simulink model "SistemaCompleto_PMSM"  (R2023b)
settings: Solver=VariableStepAuto  StartTime=0.0  StopTime=2  RelTol=1e-3
PostLoadFcn:
  | parametros_sistema_completo
  | run("parametros_sistema_completo.mlx")
values from neighbouring files (symbols this model uses):
  a_cu = 3.9e-3    (= 0.0039)    [parametros_sistema_completo.m]    (also in workspace_params.mat)
  A_i = [0,  1,                          0 ... (first row only)    [analisis_estabilidad_LA.m]
  b_eq = params.b_total    [calcular_matriz_AO.m]    (also in calculo_incertidumbre_y_control.m = b_m + b_l/(r^2); parametros_sistema_completo.m = 2.19444444444e-05; workspace_params.mat = 2.19444444444e-05)
  C_ts = C_ts * (1 + tol_pct)    [calculo_incertidumbre_y_control.m]    (also in parametros_sistema_completo.m = 0.818; workspace_params.mat = 0.818)
  g = 9.80665    [parametros_sistema_completo.m]    (also in workspace_params.mat)
  J_eq = params.J_total    [calcular_matriz_AO.m]    (also in calculo_incertidumbre_y_control.m = J_m + J_l/r^2; parametros_sistema_completo.m = 1.97847222222e-05; workspace_params.mat = 3.28055555556e-05)
  k_l = m*l_cm + m_l*l_l    [calculo_incertidumbre_y_control.m]    (also in parametros_sistema_completo.m = 0.25; workspace_params.mat = 0.625)
  L_d = L_d    * (1 - tol_pct)    [calculo_incertidumbre_y_control.m]    (also in parametros_sistema_completo.m = 0.0066; workspace_params.mat = 0.0066)
  L_ls = L_ls   * (1 - tol_pct)    [calculo_incertidumbre_y_control.m]    (also in parametros_sistema_completo.m = 0.0008; workspace_params.mat = 0.0008)
  L_q = L_q    * (1 - tol_pct)    [calculo_incertidumbre_y_control.m]    (also in parametros_sistema_completo.m = 0.0058; workspace_params.mat = 0.0058)
  lambda_r = lambda_r * (1 + tol_pct)    [calculo_incertidumbre_y_control.m]    (also in parametros_sistema_completo.m = 0.016; workspace_params.mat = 0.016)
  P_p = 3    [parametros_sistema_completo.m]    (also in workspace_params.mat)
  params = struct()    [evaluar_migracion_Ids.m]    (also in parametros_sistema_completo.m; workspace_params.mat = )
  r = params.r_red    [calcular_matriz_AO.m]    (also in parametros_sistema_completo.m = 120; workspace_params.mat = 120)
  R_s_sim = R_sREF * (1 + a_cu * (T_s_sim - T_sREF))    [configurar_temperatura_516.m]
  R_sREF = R_sREF * (1 - tol_pct)    [calculo_incertidumbre_y_control.m]    (also in parametros_sistema_completo.m = 1.02; workspace_params.mat = 1.02)
  R_ts_amb = R_ts_amb * (1 - tol_pct)    [calculo_incertidumbre_y_control.m]    (also in parametros_sistema_completo.m = 146.7; workspace_params.mat = 146.7)
  T_amb = 20    [parametros_sistema_completo.m]    (also in workspace_params.mat)
  T_s = x(6)    [modulador_torque_521.m]    (also in simulacion_dinamica_516.m)
  T_sREF = 20    [parametros_sistema_completo.m]    (also in workspace_params.mat)
undefined symbols (not defined in the file or in its folder): A_T, A_theta, A_v, b_a, B_i, B_T, B_theta, B_v, C_i, C_T, C_theta, C_v, consigna_posicion, D_i, D_T, D_theta, D_v, i_ds_inicial, Is_pico, Is_rms_max, Is_rms_nom, K_e_i_m_int, K_e_tita_m, K_e_tita_m_int, K_e_w_m, K_e_w_m_int, K_p0, K_pd, K_pq, K_sa, K_sia, pos_inicial, t_rampa_acel, t_rampa_vel, V_sl_max, x0_ias, x0_ibs, x0_ics, x0_T, x0_theta
libraries: simulink_extras x8, SignalEditorBlockLib x6, eeStairGenerator x4, simulink x1
(part 4 of 7)

== system SistemaCompleto_PMSM/Modelo Global NL perfil trapezoidal aceleracion1/Controlador PID de Posicion ==
  ωm[rad/s] : Inport
  ωm*[rad/s] : Inport  Port=2
  Integrator : Integrator
  Integrator1 : Integrator
  K_sa : Gain  Gain=K_sa
  K_sia : Gain  Gain=K_sia
  Sum : Sum  Inputs=+++
  Sum1 : Sum  Inputs=-+|
  b_a : Gain  Gain=b_a
  Tm*' : Outport
  wires:
  K_sa/1 -> Sum/2
  K_sia/1 -> Sum/3
  Integrator1/1 -> Integrator/1, K_sa/1  "eθm"
  b_a/1 -> Sum/1
  Integrator/1 -> K_sia/1  "eθ/s"
  ωm[rad/s]/1 -> Sum1/1
  ωm*[rad/s]/1 -> Sum1/2
  Sum1/1 -> b_a/1, Integrator1/1  "eωm"
  Sum/1 -> Tm*'/1  "Tm*'"

== system SistemaCompleto_PMSM/Modelo Global NL perfil trapezoidal aceleracion1/Desacople de Realimentaciones Fisicas Naturales ==
  R_s : Inport
  ωm : Inport  Port=2
  i_qs : Inport  Port=3
  v_qs* : Inport  Port=4
  v_ds* : Inport  Port=5
  v_0s* : Inport  Port=6
  i_0s : Inport  Port=7
  i_ds : Inport  Port=8
  Constant : Constant  Value=lambda_r
  Gain : Gain  Gain=P_p
  Gain3 : Gain  Gain=L_q*P_p
  Gain4 : Gain  Gain=L_d
  Product{,1..4} (5 alike) : Product
  Sum : Sum  Inputs=|++
  Sum1 : Sum  Inputs=+++
  Sum2 : Sum  Inputs=+-+
  Sum3 : Sum  Inputs=++|
  v_qs [V] : Outport
  v_ds [V] : Outport  Port=2
  v_0s [V] : Outport  Port=3
  wires:
  i_ds/1 -> Product3/1, Gain4/1
  Product1/1 -> Sum1/3
  Gain/1 -> Sum1/2
  v_qs*/1 -> Sum1/1
  R_s/1 -> Product1/2, Product3/2, Product4/1
  i_qs/1 -> Product2/2, Product1/1
  Sum1/1 -> v_qs [V]/1  "v_qs [V]"
  Gain3/1 -> Sum2/2
  Product2/1 -> Gain3/1
  Product3/1 -> Sum2/3
  v_ds*/1 -> Sum2/1
  Sum2/1 -> v_ds [V]/1  "v_ds [V]"
  i_0s/1 -> Product4/2
  Product4/1 -> Sum3/2
  v_0s*/1 -> Sum3/1
  Sum3/1 -> v_0s [V]/1
  ωm/1 -> Product/1, Product2/1
  Constant/1 -> Sum/1
  Gain4/1 -> Sum/2
  Sum/1 -> Product/2
  Product/1 -> Gain/1

== system SistemaCompleto_PMSM/Modelo Global NL perfil trapezoidal aceleracion1/Modulador de Corriente ==
  i_qs : Inport
  i_qs* : Inport  Port=2
  i_ds* : Inport  Port=3
  i_ds : Inport  Port=4
  i_0s* : Inport  Port=5
  i_0s : Inport  Port=6
  Gain : Gain  Gain=K_pq
  K_p0 : Gain  Gain=K_p0
  K_pd : Gain  Gain=K_pd
  Sum : Sum  Inputs=|+-
  Sum1 : Sum  Inputs=|+-
  Sum2 : Sum  Inputs=|+-
  v_qs* : Outport
  v_ds* : Outport  Port=2
  v_0s* : Outport  Port=3
  wires:
  i_qs*/1 -> Sum/1
  K_pd/1 -> v_ds*/1
  i_0s*/1 -> Sum2/1
  Sum/1 -> Gain/1
  i_qs/1 -> Sum/2
  K_p0/1 -> v_0s*/1
  Sum1/1 -> K_pd/1
  Sum2/1 -> K_p0/1
  Gain/1 -> v_qs*/1
  i_ds*/1 -> Sum1/1
  i_ds/1 -> Sum1/2
  i_0s/1 -> Sum2/2

== system SistemaCompleto_PMSM/Modelo Global NL perfil trapezoidal aceleracion1/Modulador de Tensión no ideal espacio de estados ==
  V_c* : Inport
  V_b* : Inport  Port=2
  V_a* : Inport  Port=3
  Saturation1 : Saturate  UpperLimit=sqrt(2/3)*V_sl_max  LowerLimit=-sqrt(2/3)*V_sl_max  ZeroCross=off
  Saturation2 : Saturate  UpperLimit=sqrt(2/3)*V_sl_max  LowerLimit=-sqrt(2/3)*V_sl_max  ZeroCross=off
  Saturation3 : Saturate  UpperLimit=sqrt(2/3)*V_sl_max  LowerLimit=-sqrt(2/3)*V_sl_max  ZeroCross=off
  State-Space : StateSpace  A=A_v  B=B_v  C=C_v  D=D_v  InitialCondition=[0;0]
  State-Space1 : StateSpace  A=A_v  B=B_v  C=C_v  D=D_v  InitialCondition=[0;0]
  State-Space2 : StateSpace  A=A_v  B=B_v  C=C_v  D=D_v  InitialCondition=[0;0]
  V_a : Outport
  V_b : Outport  Port=2
  V_c : Outport  Port=3
  wires:
  V_b*/1 -> State-Space2/1
  V_a*/1 -> State-Space/1
  V_c*/1 -> State-Space1/1
  Saturation2/1 -> V_a/1  "V_a* [V]"
  Saturation3/1 -> V_c/1  "V_c* [V]"
  Saturation1/1 -> V_b/1  "V_b* [V]"
  State-Space/1 -> Saturation2/1
  State-Space2/1 -> Saturation1/1
  State-Space1/1 -> Saturation3/1

== system SistemaCompleto_PMSM/Modelo Global NL perfil trapezoidal aceleracion1/Modulador de Torque ==
  ωm[rad/s] : Inport
  θm [rad] : Inport  Port=2
  T_m*'[N.m] : Inport  Port=3
  i_ds [A] : Inport  Port=4
  Constant : Constant  Value=lambda_r
  Gain : Gain  Gain=3/2*P_p
  Gain1 : Gain  Gain=L_d-L_q
  Gain2 : Gain  Gain=1/r
  Gain3 : Gain  Gain=k_l*g/r
  Gain4 : Gain  Gain=b_eq
  Product1 : Product  Inputs=*/
  Saturation : Saturate  UpperLimit=Is_pico  LowerLimit=-Is_pico  ZeroCross=off
  Sin : Trigonometry
  Sum : Sum  Inputs=|++
  Sum1 : Sum  Inputs=+++
  i_qs* : Outport
  wires:
  i_ds [A]/1 -> Gain1/1
  Constant/1 -> Sum/1
  Gain1/1 -> Sum/2
  Sum/1 -> Gain/1
  Gain/1 -> Product1/2
  θm [rad]/1 -> Gain2/1
  Gain2/1 -> Sin/1
  Sin/1 -> Gain3/1
  Gain3/1 -> Sum1/3
  Gain4/1 -> Sum1/2
  ωm[rad/s]/1 -> Gain4/1
  T_m*'[N.m]/1 -> Sum1/1
  Sum1/1 -> Product1/1
  Product1/1 -> Saturation/1
  Saturation/1 -> i_qs*/1

== system SistemaCompleto_PMSM/Modelo Global NL perfil trapezoidal aceleracion1/Observador de Estado de velocidad  ==
  θ : Inport
  Te*' : Inport  Port=2
  Gain : Gain  Gain=K_e_i_m_int
  Gain1 : Gain  Gain=K_e_tita_m_int
  Gain7 : Gain  Gain=K_e_w_m_int
  Gain8 : Gain  Gain=1/J_eq
  Integrator : Integrator
  Integrator1 : Integrator
  Integrator2 : Integrator
  Sum1 : Sum  Inputs=|+-
  Sum2 : Sum  Inputs=+++
  Sum3 : Sum  Inputs=++|
  ω~ : Outport
  wires:
  Gain1/1 -> Sum3/2
  Integrator/1 -> ω~/1, Sum3/1  "ω~"
  Sum1/1 -> Gain1/1, Gain7/1, Integrator2/1  "e(t)"
  Integrator1/1 -> Sum1/2  "θ~"
  Gain7/1 -> Sum2/3
  Sum2/1 -> Integrator/1  "dω~/dt"
  Gain8/1 -> Sum2/1
  Sum3/1 -> Integrator1/1  "dθ~/dt"
  θ/1 -> Sum1/1
  Integrator2/1 -> Gain/1
  Te*'/1 -> Gain8/1
  Gain/1 -> Sum2/2

== system SistemaCompleto_PMSM/Modelo Global NL perfil trapezoidal aceleracion1/Planta ==
  Tld[N.m] : Inport
  V_a [V] : Inport  Port=2
  V_b [V] : Inport  Port=3
  V_c [V] : Inport  Port=4
  Gain : Gain  Gain=P_p
  Gain2 : Gain  Gain=1/r
  Gain3 : Gain  Gain=k_l/r
  Gain4 : Gain  Gain=b_eq
  Scope{,1..6} (7 alike) : Scope
  Sin : Trigonometry
  Subsistema Electromagnetico : Subsystem
  Subsistema Mecanico : Subsystem
  Subsistema Térmico : Subsystem
  Sum1 : Sum  Inputs=+--
  TI de Park : Subsystem
  Transformacion de Park : Subsystem
  θm [rad] : Outport
  ωm[rad/s] : Outport  Port=2
  i_a [A] : Outport  Port=3
  i_b [A] : Outport  Port=4
  i_c [A] : Outport  Port=5
  T_s [°C] : Outport  Port=6
  T_m : Outport  Port=7
  T_neto : Outport  Port=8
  R_s : Outport  Port=9
  wires:
  Subsistema Térmico/1(R_s) -> R_s/1, Subsistema Electromagnetico/5(R_s(T(t)))
  Subsistema Electromagnetico/3(i_0s) -> TI de Park/3(f_0), Scope4/1, Subsistema Térmico/3(i_0s2)
  Transformacion de Park/3(f_0) -> Subsistema Electromagnetico/3(v_0s)
  Subsistema Mecanico/2(ωm(t)) -> Subsistema Electromagnetico/4(ωm), ωm[rad/s]/1, Gain4/1, Scope/1  "wm"
  Subsistema Electromagnetico/1(i_qs) -> TI de Park/1(f_q), Scope2/1, Subsistema Térmico/1(i_qs2)
  Subsistema Electromagnetico/2(i_ds) -> TI de Park/2(f_d), Scope3/1, Subsistema Térmico/2(i_ds2)
  Transformacion de Park/1(f_q) -> Subsistema Electromagnetico/1(v_qs)
  Subsistema Térmico/2(T_s) -> T_s [°C]/1, Scope1/1  "Ts"
  Transformacion de Park/2(f_d) -> Subsistema Electromagnetico/2(v_ds)
  Tld[N.m]/1 -> Subsistema Mecanico/1(Tld(t)[N.m])
  Gain/1 -> TI de Park/4(θ_r), Transformacion de Park/4(θ_r)
  TI de Park/1(f_a) -> i_a [A]/1
  TI de Park/2(f_b) -> i_b [A]/1
  TI de Park/3(f_c) -> i_c [A]/1
  V_a [V]/1 -> Transformacion de Park/1(f_a)
  V_b [V]/1 -> Transformacion de Park/2(f_b)
  V_c [V]/1 -> Transformacion de Park/3(f_c)
  Gain2/1 -> Sin/1
  Gain3/1 -> Scope5/1, Sum1/3
  Subsistema Electromagnetico/4(T_m) -> Subsistema Mecanico/2(Tm(t)[N.m]), T_m/1, Sum1/1
  Sum1/1 -> T_neto/1
  Subsistema Mecanico/1(θm(t)) -> Gain2/1, Gain/1, θm [rad]/1
  Sin/1 -> Gain3/1
  Gain4/1 -> Scope6/1, Sum1/2

== system SistemaCompleto_PMSM/Modelo Global NL perfil trapezoidal aceleracion1/Setpoint ==
  θl*(t) : Inport
  Derivative : Derivative
  Gain7 : Gain  Gain=r
  θm* [rad] : Outport
  ωm*[rad/s] : Outport  Port=2
  wires:
  Derivative/1 -> ωm*[rad/s]/1  "ωm*[rad/s]"
  θl*(t)/1 -> Gain7/1
  Gain7/1 -> θm* [rad]/1, Derivative/1  "θm* [rad]"

== system SistemaCompleto_PMSM/Modelo Global NL perfil trapezoidal aceleracion1/T. Directa de Park ==
  f_a : Inport
  f_b : Inport  Port=2
  f_c : Inport  Port=3
  θ_r : Inport  Port=4
  Add : Sum  Inputs=+++
  Add1 : Sum  Inputs=+-
  Add2 : Sum
  Add3 : Sum  Inputs=+++
  Add4 : Sum  Inputs=+++
  Constant : Constant  Value=2/3*pi
  Constant1 : Constant  Value=2/3*pi
  Cos : Trigonometry  Operator=cos
  Cos1 : Trigonometry  Operator=cos
  Cos2 : Trigonometry  Operator=cos
  Cos3 : Trigonometry
  Cos4 : Trigonometry
  Cos5 : Trigonometry
  Gain1 : Gain  Gain=2/3
  Gain2 : Gain  Gain=2/3
  Gain3 : Gain  Gain=1/3
  Product{,1..5} (6 alike) : Product
  f_q : Outport
  f_d : Outport  Port=2
  f_0 : Outport  Port=3
  wires:
  Cos5/1 -> Product5/1
  Gain2/1 -> f_q/1
  Product5/1 -> Add3/3
  Add/1 -> Gain2/1
  θ_r/1 -> Cos3/1, Cos/1, Add1/1, Add2/1
  Cos4/1 -> Product4/1
  Cos2/1 -> Product2/1
  f_a/1 -> Add4/3, Product3/2, Product/2
  Product/1 -> Add/1
  Add1/1 -> Cos1/1, Cos4/1
  f_c/1 -> Product2/2, Product5/2, Add4/1
  Constant/1 -> Add1/2
  Constant1/1 -> Add2/2
  f_b/1 -> Product1/2, Product4/2, Add4/2
  Add2/1 -> Cos2/1, Cos5/1
  Add4/1 -> Gain3/1
  Product3/1 -> Add3/1
  Product2/1 -> Add/3
  Gain3/1 -> f_0/1
  Cos3/1 -> Product3/1
  Add3/1 -> Gain1/1
  Gain1/1 -> f_d/1
  Product1/1 -> Add/2
  Cos/1 -> Product/1
  Cos1/1 -> Product1/1
  Product4/1 -> Add3/2

== system SistemaCompleto_PMSM/Modelo Global NL perfil trapezoidal aceleracion1/T. Inversa de Park ==
  θ_r : Inport
  f_q : Inport  Port=2
  f_d : Inport  Port=3
  f_0 : Inport  Port=4
  Add : Sum  Inputs=+++
  Add1 : Sum  Inputs=+-
  Add2 : Sum
  Add3 : Sum  Inputs=+++
  Add4 : Sum  Inputs=+++
  Constant : Constant  Value=2/3*pi
  Constant1 : Constant  Value=2/3*pi
  Cos : Trigonometry  Operator=cos
  Cos1 : Trigonometry
  Cos2 : Trigonometry  Operator=cos
  Cos3 : Trigonometry  Operator=cos
  Cos4 : Trigonometry
  Cos5 : Trigonometry
  Product{,1..5} (6 alike) : Product
  f_a : Outport
  f_b : Outport  Port=2
  f_c : Outport  Port=3
  wires:
  Product4/1 -> Add3/2
  Cos1/1 -> Product1/1
  Cos/1 -> Product/1
  Product1/1 -> Add/2
  Add3/1 -> f_b/1
  Cos3/1 -> Product3/1
  Product3/1 -> Add3/1
  f_d/1 -> Product1/2, Product5/2, Product4/2
  Constant1/1 -> Add2/2
  Constant/1 -> Add1/2
  f_0/1 -> Add3/3, Add4/3, Add/3
  Add1/1 -> Cos3/1, Cos4/1
  Product/1 -> Add/1
  f_q/1 -> Product/2, Product2/2, Product3/2
  Cos4/1 -> Product4/1
  θ_r/1 -> Add2/1, Add1/1, Cos/1, Cos1/1
  Add/1 -> f_a/1
  Add4/1 -> f_c/1
  Cos2/1 -> Product2/1
  Cos5/1 -> Product5/1
  Add2/1 -> Cos5/1, Cos2/1
  Product2/1 -> Add4/1
  Product5/1 -> Add4/2

== system SistemaCompleto_PMSM/Modelo Global NL perfil trapezoidal aceleracion2/Controlador PID de Posicion ==
  ωm[rad/s] : Inport
  ωm*[rad/s] : Inport  Port=2
  Integrador Tustin : Subsystem
  Integrador Tustin1 : Subsystem
  K_sa : Gain  Gain=K_sa
  K_sia : Gain  Gain=K_sia
  Sum : Sum  Inputs=+++
  Sum1 : Sum  Inputs=-+|
  Zero-Order Hold : ZeroOrderHold  SampleTime=T_s
  Zero-Order Hold1 : ZeroOrderHold  SampleTime=T_s
  b_a : Gain  Gain=b_a
  Tm*' : Outport
  wires:
  Sum/1 -> Zero-Order Hold/1  "Tm*'"
  Sum1/1 -> Zero-Order Hold1/1  "eωm"
  ωm*[rad/s]/1 -> Sum1/2
  ωm[rad/s]/1 -> Sum1/1
  Integrador Tustin1/1(Int) -> K_sia/1  "eθ/s"
  b_a/1 -> Sum/1
  Integrador Tustin/1(Int) -> Integrador Tustin1/1(Actual), K_sa/1  "eθm"
  K_sia/1 -> Sum/3
  K_sa/1 -> Sum/2
  Zero-Order Hold/1 -> Tm*'/1
  Zero-Order Hold1/1 -> Integrador Tustin/1(Actual), b_a/1

== system SistemaCompleto_PMSM/Modelo Global NL perfil trapezoidal aceleracion2/Desacople de Realimentaciones Fisicas Naturales ==
  R_s : Inport
  ωm : Inport  Port=2
  i_qs : Inport  Port=3
  v_qs* : Inport  Port=4
  v_ds* : Inport  Port=5
  v_0s* : Inport  Port=6
  i_0s : Inport  Port=7
  i_ds : Inport  Port=8
  Constant : Constant  Value=lambda_r
  Gain : Gain  Gain=P_p
  Gain3 : Gain  Gain=L_q*P_p
  Gain4 : Gain  Gain=L_d
  Product{,1..4} (5 alike) : Product
  Sum : Sum  Inputs=|++
  Sum1 : Sum  Inputs=+++
  Sum2 : Sum  Inputs=+-+
  Sum3 : Sum  Inputs=++|
  v_qs [V] : Outport
  v_ds [V] : Outport  Port=2
  v_0s [V] : Outport  Port=3
  wires:
  Product/1 -> Gain/1
  Sum/1 -> Product/2
  Gain4/1 -> Sum/2
  Constant/1 -> Sum/1
  ωm/1 -> Product2/1, Product/1
  Sum3/1 -> v_0s [V]/1
  v_0s*/1 -> Sum3/1
  Product4/1 -> Sum3/2
  i_0s/1 -> Product4/2
  Sum2/1 -> v_ds [V]/1  "v_ds [V]"
  v_ds*/1 -> Sum2/1
  Product3/1 -> Sum2/3
  Product2/1 -> Gain3/1
  Gain3/1 -> Sum2/2
  Sum1/1 -> v_qs [V]/1  "v_qs [V]"
  i_qs/1 -> Product1/1, Product2/2
  R_s/1 -> Product4/1, Product3/2, Product1/2
  v_qs*/1 -> Sum1/1
  Gain/1 -> Sum1/2
  Product1/1 -> Sum1/3
  i_ds/1 -> Gain4/1, Product3/1

== system SistemaCompleto_PMSM/Modelo Global NL perfil trapezoidal aceleracion2/Modulador de Corriente ==
  i_qs : Inport
  i_qs* : Inport  Port=2
  i_ds* : Inport  Port=3
  i_ds : Inport  Port=4
  i_0s* : Inport  Port=5
  i_0s : Inport  Port=6
  Gain : Gain  Gain=K_pq
  K_p0 : Gain  Gain=K_p0
  K_pd : Gain  Gain=K_pd
  Sum : Sum  Inputs=|+-
  Sum1 : Sum  Inputs=|+-
  Sum2 : Sum  Inputs=|+-
  v_qs* : Outport
  v_ds* : Outport  Port=2
  v_0s* : Outport  Port=3
  wires:
  i_0s/1 -> Sum2/2
  i_ds/1 -> Sum1/2
  i_ds*/1 -> Sum1/1
  Gain/1 -> v_qs*/1
  Sum2/1 -> K_p0/1
  Sum1/1 -> K_pd/1
  K_p0/1 -> v_0s*/1
  i_qs/1 -> Sum/2
  Sum/1 -> Gain/1
  i_0s*/1 -> Sum2/1
  K_pd/1 -> v_ds*/1
  i_qs*/1 -> Sum/1

== system SistemaCompleto_PMSM/Modelo Global NL perfil trapezoidal aceleracion2/Modulador de Tensión no ideal espacio de estados ==
  V_c* : Inport
  V_b* : Inport  Port=2
  V_a* : Inport  Port=3
  Saturation1 : Saturate  UpperLimit=sqrt(2/3)*V_sl_max  LowerLimit=-sqrt(2/3)*V_sl_max  ZeroCross=off
  Saturation2 : Saturate  UpperLimit=sqrt(2/3)*V_sl_max  LowerLimit=-sqrt(2/3)*V_sl_max  ZeroCross=off
  Saturation3 : Saturate  UpperLimit=sqrt(2/3)*V_sl_max  LowerLimit=-sqrt(2/3)*V_sl_max  ZeroCross=off
  State-Space : StateSpace  A=A_v  B=B_v  C=C_v  D=D_v  InitialCondition=[0;0]
  State-Space1 : StateSpace  A=A_v  B=B_v  C=C_v  D=D_v  InitialCondition=[0;0]
  State-Space2 : StateSpace  A=A_v  B=B_v  C=C_v  D=D_v  InitialCondition=[0;0]
  V_a : Outport
  V_b : Outport  Port=2
  V_c : Outport  Port=3
  wires:
  State-Space1/1 -> Saturation3/1
  State-Space2/1 -> Saturation1/1
  State-Space/1 -> Saturation2/1
  Saturation1/1 -> V_b/1  "V_b* [V]"
  Saturation3/1 -> V_c/1  "V_c* [V]"
  Saturation2/1 -> V_a/1  "V_a* [V]"
  V_c*/1 -> State-Space1/1
  V_a*/1 -> State-Space/1
  V_b*/1 -> State-Space2/1

== system SistemaCompleto_PMSM/Modelo Global NL perfil trapezoidal aceleracion2/Modulador de Torque ==
  ωm[rad/s] : Inport
  θm [rad] : Inport  Port=2
  T_m*'[N.m] : Inport  Port=3
  i_ds [A] : Inport  Port=4
  g[m/s2] : Inport  Port=5
  Constant : Constant  Value=lambda_r
  Gain : Gain  Gain=3/2*P_p
  Gain1 : Gain  Gain=L_d-L_q
  Gain2 : Gain  Gain=1/r
  Gain3 : Gain  Gain=k_l/r
  Gain4 : Gain  Gain=b_eq
  Product : Product
  Product1 : Product  Inputs=*/
  Saturation : Saturate  UpperLimit=Is_pico  LowerLimit=-Is_pico  ZeroCross=off
  Sin : Trigonometry
  Sum : Sum  Inputs=|++
  Sum1 : Sum  Inputs=+++
  i_qs* : Outport
  wires:
  Gain3/1 -> Product/1
  Sin/1 -> Gain3/1
  ωm[rad/s]/1 -> Gain4/1
  Product1/1 -> Saturation/1
  Sum/1 -> Gain/1
  Gain4/1 -> Sum1/2
  Saturation/1 -> i_qs*/1
  Gain2/1 -> Sin/1
  Constant/1 -> Sum/1
  Gain1/1 -> Sum/2
  Sum1/1 -> Product1/1
  T_m*'[N.m]/1 -> Sum1/1
  g[m/s2]/1 -> Product/2
  Gain/1 -> Product1/2
  Product/1 -> Sum1/3
  i_ds [A]/1 -> Gain1/1
  θm [rad]/1 -> Gain2/1

== system SistemaCompleto_PMSM/Modelo Global NL perfil trapezoidal aceleracion2/Observador de Estado de velocidad  ==
  θ : Inport
  Te*' : Inport  Port=2
  Gain : Gain  Gain=K_e_i_m_int
  Gain1 : Gain  Gain=K_e_tita_m_int
  Gain7 : Gain  Gain=K_e_w_m_int
  Gain8 : Gain  Gain=1/J_eq
  Integrador Tustin1 : Subsystem
  Integrador Tustin2 : Subsystem
  Integrador Tustin3 : Subsystem
  Sum1 : Sum  Inputs=|+-
  Sum2 : Sum  Inputs=+++
  Sum3 : Sum  Inputs=++|
  Zero-Order Hold : ZeroOrderHold  SampleTime=T_s
  Zero-Order Hold1 : ZeroOrderHold  SampleTime=T_s
  Zero-Order Hold2 : ZeroOrderHold  SampleTime=T_s
  ω~ : Outport
  wires:
  Gain/1 -> Sum2/2
  Te*'/1 -> Zero-Order Hold1/1
  Integrador Tustin2/1(Int) -> Gain/1
  θ/1 -> Zero-Order Hold2/1
  Sum3/1 -> Integrador Tustin3/1(Actual)  "dθ~/dt"
  Gain8/1 -> Sum2/1
  Sum2/1 -> Integrador Tustin1/1(Actual)  "dω~/dt"
  Gain7/1 -> Sum2/3
  Integrador Tustin3/1(Int) -> Sum1/2  "θ~"
  Sum1/1 -> Integrador Tustin2/1(Actual), Gain7/1, Gain1/1  "e(t)"
  Integrador Tustin1/1(Int) -> Sum3/1, Zero-Order Hold/1  "ω~"
  Gain1/1 -> Sum3/2
  Zero-Order Hold/1 -> ω~/1
  Zero-Order Hold1/1 -> Gain8/1
  Zero-Order Hold2/1 -> Sum1/1

== system SistemaCompleto_PMSM/Modelo Global NL perfil trapezoidal aceleracion2/Planta ==
  Tld[N.m] : Inport
  V_a [V] : Inport  Port=2
  V_b [V] : Inport  Port=3
  V_c [V] : Inport  Port=4
  g[m/s2] : Inport  Port=5
  Gain : Gain  Gain=P_p
  Gain2 : Gain  Gain=1/r
  Gain3 : Gain  Gain=k_l/r
  Gain4 : Gain  Gain=b_eq
  Scope{,1..6} (7 alike) : Scope
  Sin : Trigonometry
  Subsistema Electromagnetico : Subsystem
  Subsistema Mecanico : Subsystem
  Subsistema Térmico : Subsystem
  Sum1 : Sum  Inputs=+--
  TI de Park : Subsystem
  Transformacion de Park : Subsystem
  θm [rad] : Outport
  ωm[rad/s] : Outport  Port=2
  i_a [A] : Outport  Port=3
  i_b [A] : Outport  Port=4
  i_c [A] : Outport  Port=5
  T_s [°C] : Outport  Port=6
  T_m : Outport  Port=7
  T_neto : Outport  Port=8
  R_s : Outport  Port=9
  wires:
  Gain4/1 -> Sum1/2, Scope6/1
  Sin/1 -> Gain3/1
  ? -> θm [rad]/1, Gain/1, Gain2/1
  Sum1/1 -> T_neto/1
  Subsistema Electromagnetico/4(T_m) -> Sum1/1, T_m/1
  Gain3/1 -> Sum1/3, Scope5/1
  Gain2/1 -> Sin/1
  V_c [V]/1 -> Transformacion de Park/3(f_c)
  V_b [V]/1 -> Transformacion de Park/2(f_b)
  V_a [V]/1 -> Transformacion de Park/1(f_a)
  TI de Park/3(f_c) -> i_c [A]/1
  TI de Park/2(f_b) -> i_b [A]/1
  TI de Park/1(f_a) -> i_a [A]/1
  Gain/1 -> Transformacion de Park/4(θ_r), TI de Park/4(θ_r)
  Tld[N.m]/1 -> ?
  Transformacion de Park/2(f_d) -> Subsistema Electromagnetico/2(v_ds)
  Subsistema Térmico/2(T_s) -> Scope1/1, T_s [°C]/1  "Ts"
  Transformacion de Park/1(f_q) -> Subsistema Electromagnetico/1(v_qs)
  Subsistema Electromagnetico/2(i_ds) -> Subsistema Térmico/2(i_ds2), Scope3/1, TI de Park/2(f_d)
  Subsistema Electromagnetico/1(i_qs) -> Subsistema Térmico/1(i_qs2), Scope2/1, TI de Park/1(f_q)
  ? -> Scope/1, Gain4/1, ωm[rad/s]/1, Subsistema Electromagnetico/4(ωm)  "wm"
  Transformacion de Park/3(f_0) -> Subsistema Electromagnetico/3(v_0s)
  Subsistema Electromagnetico/3(i_0s) -> Subsistema Térmico/3(i_0s2), Scope4/1, TI de Park/3(f_0)
  Subsistema Térmico/1(R_s) -> Subsistema Electromagnetico/5(R_s(T(t))), R_s/1
  g[m/s2]/1 -> Subsistema Mecanico/3(g [m/s2])

== system SistemaCompleto_PMSM/Modelo Global NL perfil trapezoidal aceleracion2/Setpoint ==
  θl*(t) : Inport
  Derivative : Derivative
  Gain7 : Gain  Gain=r
  θm* [rad] : Outport
  ωm*[rad/s] : Outport  Port=2
  wires:
  Gain7/1 -> Derivative/1, θm* [rad]/1  "θm* [rad]"
  θl*(t)/1 -> Gain7/1
  Derivative/1 -> ωm*[rad/s]/1  "ωm*[rad/s]"

== system SistemaCompleto_PMSM/Modelo Global NL perfil trapezoidal aceleracion2/T. Directa de Park ==
  f_a : Inport
  f_b : Inport  Port=2
  f_c : Inport  Port=3
  θ_r : Inport  Port=4
  Add : Sum  Inputs=+++
  Add1 : Sum  Inputs=+-
  Add2 : Sum
  Add3 : Sum  Inputs=+++
  Add4 : Sum  Inputs=+++
  Constant : Constant  Value=2/3*pi
  Constant1 : Constant  Value=2/3*pi
  Cos : Trigonometry  Operator=cos
  Cos1 : Trigonometry  Operator=cos
  Cos2 : Trigonometry  Operator=cos
  Cos3 : Trigonometry
  Cos4 : Trigonometry
  Cos5 : Trigonometry
  Gain1 : Gain  Gain=2/3
  Gain2 : Gain  Gain=2/3
  Gain3 : Gain  Gain=1/3
  Product{,1..5} (6 alike) : Product
  f_q : Outport
  f_d : Outport  Port=2
  f_0 : Outport  Port=3
  wires:
  Product4/1 -> Add3/2
  Cos1/1 -> Product1/1
  Cos/1 -> Product/1
  Product1/1 -> Add/2
  Gain1/1 -> f_d/1
  Add3/1 -> Gain1/1
  Cos3/1 -> Product3/1
  Gain3/1 -> f_0/1
  Product2/1 -> Add/3
  Product3/1 -> Add3/1
  Add4/1 -> Gain3/1
  Add2/1 -> Cos5/1, Cos2/1
  f_b/1 -> Add4/2, Product4/2, Product1/2
  Constant1/1 -> Add2/2
  Constant/1 -> Add1/2
  f_c/1 -> Add4/1, Product5/2, Product2/2
  Add1/1 -> Cos4/1, Cos1/1
  Product/1 -> Add/1
  f_a/1 -> Product/2, Product3/2, Add4/3
  Cos2/1 -> Product2/1
  Cos4/1 -> Product4/1
  θ_r/1 -> Add2/1, Add1/1, Cos/1, Cos3/1
  Add/1 -> Gain2/1
  Product5/1 -> Add3/3
  Gain2/1 -> f_q/1
  Cos5/1 -> Product5/1

== system SistemaCompleto_PMSM/Modelo Global NL perfil trapezoidal aceleracion2/T. Inversa de Park ==
  θ_r : Inport
  f_q : Inport  Port=2
  f_d : Inport  Port=3
  f_0 : Inport  Port=4
  Add : Sum  Inputs=+++
  Add1 : Sum  Inputs=+-
  Add2 : Sum
  Add3 : Sum  Inputs=+++
  Add4 : Sum  Inputs=+++
  Constant : Constant  Value=2/3*pi
  Constant1 : Constant  Value=2/3*pi
  Cos : Trigonometry  Operator=cos
  Cos1 : Trigonometry
  Cos2 : Trigonometry  Operator=cos
  Cos3 : Trigonometry  Operator=cos
  Cos4 : Trigonometry
  Cos5 : Trigonometry
  Product{,1..5} (6 alike) : Product
  f_a : Outport
  f_b : Outport  Port=2
  f_c : Outport  Port=3
  wires:
  Product5/1 -> Add4/2
  Product2/1 -> Add4/1
  Add2/1 -> Cos2/1, Cos5/1
  Cos5/1 -> Product5/1
  Cos2/1 -> Product2/1
  Add4/1 -> f_c/1
  Add/1 -> f_a/1
  θ_r/1 -> Cos1/1, Cos/1, Add1/1, Add2/1
  Cos4/1 -> Product4/1
  f_q/1 -> Product3/2, Product2/2, Product/2
  Product/1 -> Add/1
  Add1/1 -> Cos4/1, Cos3/1
  f_0/1 -> Add/3, Add4/3, Add3/3
  Constant/1 -> Add1/2
  Constant1/1 -> Add2/2
  f_d/1 -> Product4/2, Product5/2, Product1/2
  Product3/1 -> Add3/1
  Cos3/1 -> Product3/1
  Add3/1 -> f_b/1
  Product1/1 -> Add/2
  Cos/1 -> Product/1
  Cos1/1 -> Product1/1
  Product4/1 -> Add3/2

== system SistemaCompleto_PMSM/Modelo Global NL Retroalimentado/Modulador de Tensión Ganancia unitaria ==
  V_a* : Inport
  V_b* : Inport  Port=2
  V_c* : Inport  Port=3
  Gain : Gain
  Gain1 : Gain
  Gain2 : Gain
  V_a : Outport
  V_b : Outport  Port=2
  V_c : Outport  Port=3
  wires:
  V_b*/1 -> Gain/1
  V_a*/1 -> Gain2/1
  V_c*/1 -> Gain1/1
  Gain/1 -> V_b/1
  Gain2/1 -> V_a/1
  Gain1/1 -> V_c/1

== system SistemaCompleto_PMSM/Modelo Global NL Retroalimentado/Planta ==
  Tld[N.m] : Inport
  V_a [V] : Inport  Port=2
  V_b [V] : Inport  Port=3
  V_c [V] : Inport  Port=4
  Constant : Constant  Value=R_s_sim
  Gain : Gain  Gain=P_p
  Scope : Scope
  Scope1 : Scope
  Subsistema Electromagnetico : Subsystem
  Subsistema Mecanico : Subsystem
  Subsistema Térmico : Subsystem
  TI de Park : Subsystem
  Transformacion de Park : Subsystem
  θm [rad] : Outport
  ωm[rad/s] : Outport  Port=2
  i_a [A] : Outport  Port=3
  i_b [A] : Outport  Port=4
  i_c [A] : Outport  Port=5
  T_s [°C] : Outport  Port=6
  T_m : Outport  Port=7
  wires:
  Subsistema Electromagnetico/3(i_0s) -> TI de Park/3(f_0), Subsistema Térmico/3(i_0s2)
  Subsistema Electromagnetico/4(T_m) -> T_m/1, Subsistema Mecanico/2(Tm(t)[N.m])
  Transformacion de Park/3(f_0) -> Subsistema Electromagnetico/3(v_0s)
  Subsistema Mecanico/2(ωm(t)) -> Subsistema Electromagnetico/4(ωm), Scope/1, ωm[rad/s]/1  "wm"
  Subsistema Electromagnetico/1(i_qs) -> TI de Park/1(f_q), Subsistema Térmico/1(i_qs2)
  Subsistema Electromagnetico/2(i_ds) -> TI de Park/2(f_d), Subsistema Térmico/2(i_ds2)
  Transformacion de Park/1(f_q) -> Subsistema Electromagnetico/1(v_qs)
  Subsistema Térmico/2(T_s) -> T_s [°C]/1, Scope1/1  "Ts"
  Transformacion de Park/2(f_d) -> Subsistema Electromagnetico/2(v_ds)
  Subsistema Mecanico/1(θm(t)) -> Gain/1, θm [rad]/1
  Tld[N.m]/1 -> Subsistema Mecanico/1(Tld(t)[N.m])
  Gain/1 -> TI de Park/4(θ_r), Transformacion de Park/4(θ_r)
  TI de Park/1(f_a) -> i_a [A]/1
  TI de Park/2(f_b) -> i_b [A]/1
  TI de Park/3(f_c) -> i_c [A]/1
  V_a [V]/1 -> Transformacion de Park/1(f_a)
  V_b [V]/1 -> Transformacion de Park/2(f_b)
  V_c [V]/1 -> Transformacion de Park/3(f_c)
  Subsistema Térmico/1(R_s) -> Subsistema Electromagnetico/5(R_s)

== system SistemaCompleto_PMSM/Modelo Global NL Retroalimentado/T. Directa de Park ==
  f_a : Inport
  f_b : Inport  Port=2
  f_c : Inport  Port=3
  θ_r : Inport  Port=4
  Add : Sum  Inputs=+++
  Add1 : Sum  Inputs=+-
  Add2 : Sum
  Add3 : Sum  Inputs=+++
  Add4 : Sum  Inputs=+++
  Constant : Constant  Value=2/3*pi
  Constant1 : Constant  Value=2/3*pi
  Cos : Trigonometry  Operator=cos
  Cos1 : Trigonometry  Operator=cos
  Cos2 : Trigonometry  Operator=cos
  Cos3 : Trigonometry
  Cos4 : Trigonometry
  Cos5 : Trigonometry
  Gain1 : Gain  Gain=2/3
  Gain2 : Gain  Gain=2/3
  Gain3 : Gain  Gain=1/3
  Product{,1..5} (6 alike) : Product
  f_q : Outport
  f_d : Outport  Port=2
  f_0 : Outport  Port=3
  wires:
  Cos5/1 -> Product5/1
  Gain2/1 -> f_q/1
  Product5/1 -> Add3/3
  Add/1 -> Gain2/1
  θ_r/1 -> Cos3/1, Cos/1, Add1/1, Add2/1
  Cos4/1 -> Product4/1
  Cos2/1 -> Product2/1
  f_a/1 -> Add4/3, Product3/2, Product/2
  Product/1 -> Add/1
  Add1/1 -> Cos1/1, Cos4/1
  f_c/1 -> Product2/2, Product5/2, Add4/1
  Constant/1 -> Add1/2
  Constant1/1 -> Add2/2
  f_b/1 -> Product1/2, Product4/2, Add4/2
  Add2/1 -> Cos2/1, Cos5/1
  Add4/1 -> Gain3/1
  Product3/1 -> Add3/1
  Product2/1 -> Add/3
  Gain3/1 -> f_0/1
  Cos3/1 -> Product3/1
  Add3/1 -> Gain1/1
  Gain1/1 -> f_d/1
  Product1/1 -> Add/2
  Cos/1 -> Product/1
  Cos1/1 -> Product1/1
  Product4/1 -> Add3/2

== system SistemaCompleto_PMSM/Modelo Global NL Retroalimentado/T. Inversa de Park ==
  f_q : Inport
  f_d : Inport  Port=2
  f_0 : Inport  Port=3
  θ_r : Inport  Port=4
  Add : Sum  Inputs=+++
  Add1 : Sum  Inputs=+-
  Add2 : Sum
  Add3 : Sum  Inputs=+++
  Add4 : Sum  Inputs=+++
  Constant : Constant  Value=2/3*pi
  Constant1 : Constant  Value=2/3*pi
  Cos : Trigonometry  Operator=cos
  Cos1 : Trigonometry
  Cos2 : Trigonometry  Operator=cos
  Cos3 : Trigonometry  Operator=cos
  Cos4 : Trigonometry
  Cos5 : Trigonometry
  Product{,1..5} (6 alike) : Product
  f_a : Outport
  f_b : Outport  Port=2
  f_c : Outport  Port=3
  wires:
  Product4/1 -> Add3/2
  Cos1/1 -> Product1/1
  Cos/1 -> Product/1
  Product1/1 -> Add/2
  Add3/1 -> f_b/1
  Cos3/1 -> Product3/1
  Product3/1 -> Add3/1
  f_d/1 -> Product1/2, Product5/2, Product4/2
  Constant1/1 -> Add2/2
  Constant/1 -> Add1/2
  f_0/1 -> Add3/3, Add4/3, Add/3
  Add1/1 -> Cos3/1, Cos4/1
  Product/1 -> Add/1
  f_q/1 -> Product/2, Product2/2, Product3/2
  Cos4/1 -> Product4/1
  θ_r/1 -> Add2/1, Add1/1, Cos/1, Cos1/1
  Add/1 -> f_a/1
  Add4/1 -> f_c/1
  Cos2/1 -> Product2/1
  Cos5/1 -> Product5/1
  Add2/1 -> Cos5/1, Cos2/1
  Product2/1 -> Add4/1
  Product5/1 -> Add4/2

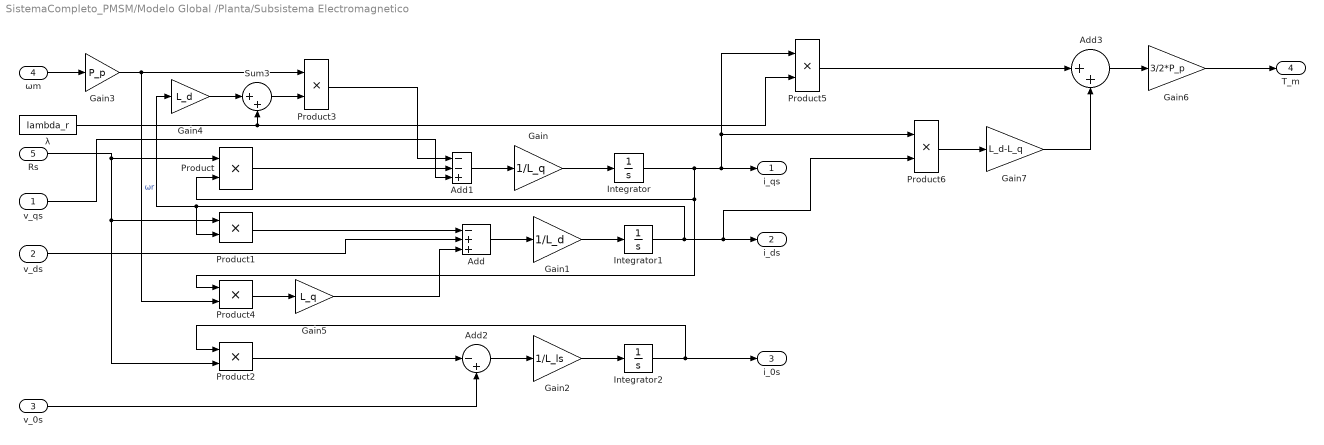
== system SistemaCompleto_PMSM/Modelo Global /Planta/Subsistema Electromagnetico ==
  v_qs : Inport
  v_ds : Inport  Port=2
  v_0s : Inport  Port=3
  ωm : Inport  Port=4
  Rs : Inport  Port=5
  Add : Sum  Inputs=-++
  Add1 : Sum  Inputs=--+
  Add2 : Sum  Inputs=|-+
  Add3 : Sum  Inputs=|++
  Gain : Gain  Gain=1/L_q
  Gain1 : Gain  Gain=1/L_d
  Gain2 : Gain  Gain=1/L_ls
  Gain3 : Gain  Gain=P_p
  Gain4 : Gain  Gain=L_d
  Gain5 : Gain  Gain=L_q
  Gain6 : Gain  Gain=3/2*P_p
  Gain7 : Gain  Gain=L_d-L_q
  Integrator : Integrator
  Integrator1 : Integrator  InitialCondition=i_ds_inicial
  Integrator2 : Integrator
  Product{,1..6} (7 alike) : Product
  Sum3 : Sum  Inputs=|++
  λ : Constant  Value=lambda_r
  i_qs : Outport
  i_ds : Outport  Port=2
  i_0s : Outport  Port=3
  T_m : Outport  Port=4
  wires:
  v_0s/1 -> Add2/2
  Gain5/1 -> Add/3
  Gain3/1 -> Product4/2, Product3/1  "ωr"
  Integrator/1 -> Product4/1, Product/2, i_qs/1, Product5/1, Product6/1
  v_qs/1 -> Add1/3
  Rs/1 -> Product2/2, Product1/1, Product/1
  Gain4/1 -> Sum3/1
  Product1/1 -> Add/1
  Integrator2/1 -> i_0s/1, Product2/1
  Sum3/1 -> Product3/2
  Integrator1/1 -> Gain4/1, Product1/2, i_ds/1, Product6/2
  Product/1 -> Add1/2
  Product4/1 -> Gain5/1
  ωm/1 -> Gain3/1
  Add3/1 -> Gain6/1
  Gain/1 -> Integrator/1
  Gain6/1 -> T_m/1
  Product2/1 -> Add2/1
  λ/1 -> Sum3/2, Product5/2
  Gain1/1 -> Integrator1/1
  Add/1 -> Gain1/1
  Add1/1 -> Gain/1
  Product6/1 -> Gain7/1
  Product3/1 -> Add1/1
  Gain2/1 -> Integrator2/1
  Gain7/1 -> Add3/2
  v_ds/1 -> Add/2
  Add2/1 -> Gain2/1
  Product5/1 -> Add3/1

== system SistemaCompleto_PMSM/Modelo Global /Planta/Subsistema Mecanico ==
  Tld(t)[N.m] : Inport
  Tm(t)[N.m] : Inport  Port=2
  1/J_eq[kg.m2] : Gain  Gain=1/J_eq
  Gain : Gain  Gain=1/r
  Gain1 : Gain  Gain=1/r
  Integrator : Integrator
  Integrator1 : Integrator
  Sin : Trigonometry
  Sum : Sum  Inputs=-+-
  Sum1 : Sum
  "[N.m/rad]" : Gain  Gain=g*k_l
  b_eq[N.m/rad/s] : Gain  Gain=b_eq
  θm(t) : Outport
  ωm(t) : Outport  Port=2
  wires:
  Gain1/1 -> Sin/1
  Sin/1 -> "[N.m/rad]"/1  "θm[rad]"
  Integrator1/1 -> Integrator/1, ωm(t)/1, b_eq[N.m/rad/s]/1  "ωm[rad/s]"
  Tld(t)[N.m]/1 -> Sum1/1
  b_eq[N.m/rad/s]/1 -> Sum/3
  1/J_eq[kg.m2]/1 -> Integrator1/1  "dω/dt [rad/s^2]"
  Gain/1 -> Sum/1
  "[N.m/rad]"/1 -> Sum1/2
  Integrator/1 -> θm(t)/1, Gain1/1  "θm[rad]"
  Sum/1 -> 1/J_eq[kg.m2]/1
  Tm(t)[N.m]/1 -> Sum/2
  Sum1/1 -> Gain/1

== system SistemaCompleto_PMSM/Modelo Global /Planta/Subsistema Térmico ==
  i_qs2 : Inport
  i_ds2 : Inport  Port=2
  i_0s2 : Inport  Port=3
  Add : Sum  Inputs=+-
  Add1 : Sum
  Add2 : Sum  Inputs=+++
  Add3 : Sum  Inputs=+-
  Add4 : Sum  Inputs=-+
  Constant : Constant  Value=T_sREF
  Constant1 : Constant
  Constant2 : Constant  Value=T_amb
  Gain : Gain  Gain=R_sREF
  Gain1 : Gain  Gain=a_cu
  Gain2 : Gain  Gain=3/2
  Gain3 : Gain  Gain=2
  Gain4 : Gain  Gain=1/C_ts
  Gain5 : Gain  Gain=1/R_ts_amb
  Integrator : Integrator  InitialCondition=20
  Product : Product
  Square : Math  Operator=square  OutDataTypeStr=double
  Square1 : Math  Operator=square
  Square2 : Math  Operator=square
  R_s : Outport
  T_s : Outport  Port=2
  wires:
  Constant1/1 -> Add1/2
  Constant/1 -> Add/2
  i_qs2/1 -> Square/1
  Gain/1 -> R_s/1, Product/1
  Square/1 -> Add2/1
  Add2/1 -> Gain2/1
  Constant2/1 -> Add4/1
  i_ds2/1 -> Square1/1
  Gain5/1 -> Add3/2
  Integrator/1 -> Add4/2, T_s/1, Add/1  "T_s"
  Add1/1 -> Gain/1
  i_0s2/1 -> Square2/1
  Square1/1 -> Add2/2
  Product/1 -> Add3/1  "Ps_Perd"
  Gain2/1 -> Product/2
  Add/1 -> Gain1/1
  Square2/1 -> Gain3/1
  Gain1/1 -> Add1/1
  Add3/1 -> Gain4/1
  Add4/1 -> Gain5/1
  Gain3/1 -> Add2/3
  Gain4/1 -> Integrator/1

== system SistemaCompleto_PMSM/Modelo Global /Planta/TI de Park ==
  f_q : Inport
  f_d : Inport  Port=2
  f_0 : Inport  Port=3
  θ_r : Inport  Port=4
  Add : Sum  Inputs=+++
  Add1 : Sum  Inputs=+-
  Add2 : Sum
  Add3 : Sum  Inputs=+++
  Add4 : Sum  Inputs=+++
  Constant : Constant  Value=2/3*pi
  Constant1 : Constant  Value=2/3*pi
  Cos : Trigonometry  Operator=cos
  Cos1 : Trigonometry
  Cos2 : Trigonometry  Operator=cos
  Cos3 : Trigonometry  Operator=cos
  Cos4 : Trigonometry
  Cos5 : Trigonometry
  Product{,1..5} (6 alike) : Product
  f_a : Outport
  f_b : Outport  Port=2
  f_c : Outport  Port=3
  wires:
  Product4/1 -> Add3/2
  Cos1/1 -> Product1/1
  Cos/1 -> Product/1
  Product1/1 -> Add/2
  Add3/1 -> f_b/1
  Cos3/1 -> Product3/1
  Product3/1 -> Add3/1
  f_d/1 -> Product1/2, Product5/2, Product4/2
  Constant1/1 -> Add2/2
  Constant/1 -> Add1/2
  f_0/1 -> Add3/3, Add4/3, Add/3
  Add1/1 -> Cos3/1, Cos4/1
  Product/1 -> Add/1
  f_q/1 -> Product/2, Product2/2, Product3/2
  Cos4/1 -> Product4/1
  θ_r/1 -> Add2/1, Add1/1, Cos/1, Cos1/1
  Add/1 -> f_a/1
  Add4/1 -> f_c/1
  Cos2/1 -> Product2/1
  Cos5/1 -> Product5/1
  Add2/1 -> Cos5/1, Cos2/1
  Product2/1 -> Add4/1
  Product5/1 -> Add4/2

== system SistemaCompleto_PMSM/Modelo Global /Planta/Transformacion de Park ==
  f_a : Inport
  f_b : Inport  Port=2
  f_c : Inport  Port=3
  θ_r : Inport  Port=4
  Add : Sum  Inputs=+++
  Add1 : Sum  Inputs=+-
  Add2 : Sum
  Add3 : Sum  Inputs=+++
  Add4 : Sum  Inputs=+++
  Constant : Constant  Value=2/3*pi
  Constant1 : Constant  Value=2/3*pi
  Cos : Trigonometry  Operator=cos
  Cos1 : Trigonometry  Operator=cos
  Cos2 : Trigonometry  Operator=cos
  Cos3 : Trigonometry
  Cos4 : Trigonometry
  Cos5 : Trigonometry
  Gain1 : Gain  Gain=2/3
  Gain2 : Gain  Gain=2/3
  Gain3 : Gain  Gain=1/3
  Product{,1..5} (6 alike) : Product
  f_q : Outport
  f_d : Outport  Port=2
  f_0 : Outport  Port=3
  wires:
  Cos5/1 -> Product5/1
  Gain2/1 -> f_q/1
  Product5/1 -> Add3/3
  Add/1 -> Gain2/1
  θ_r/1 -> Cos3/1, Cos/1, Add1/1, Add2/1
  Cos4/1 -> Product4/1
  Cos2/1 -> Product2/1
  f_a/1 -> Add4/3, Product3/2, Product/2
  Product/1 -> Add/1
  Add1/1 -> Cos1/1, Cos4/1
  f_c/1 -> Product2/2, Product5/2, Add4/1
  Constant/1 -> Add1/2
  Constant1/1 -> Add2/2
  f_b/1 -> Product1/2, Product4/2, Add4/2
  Add2/1 -> Cos2/1, Cos5/1
  Add4/1 -> Gain3/1
  Product3/1 -> Add3/1
  Product2/1 -> Add/3
  Gain3/1 -> f_0/1
  Cos3/1 -> Product3/1
  Add3/1 -> Gain1/1
  Gain1/1 -> f_d/1
  Product1/1 -> Add/2
  Cos/1 -> Product/1
  Cos1/1 -> Product1/1
  Product4/1 -> Add3/2

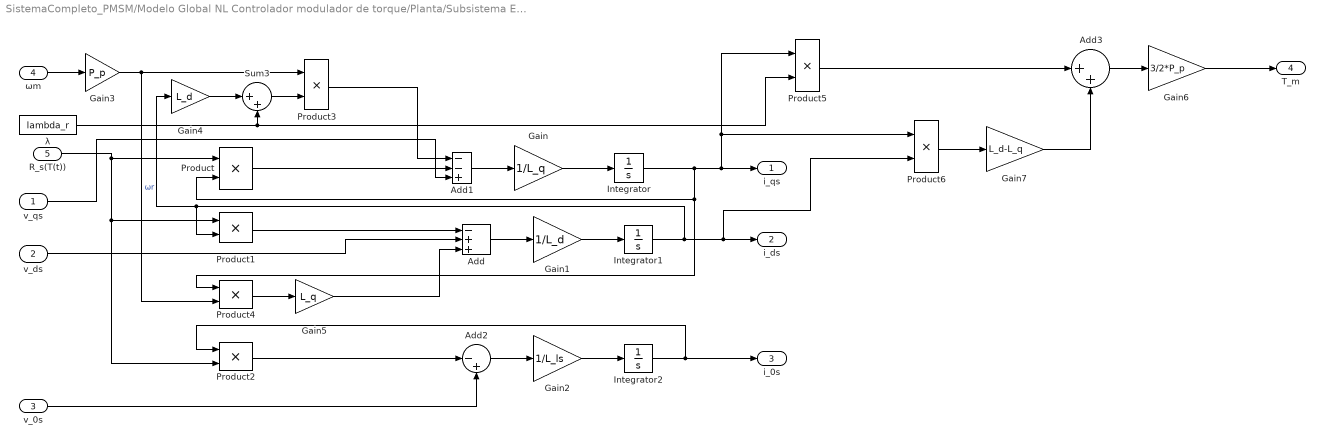
== system SistemaCompleto_PMSM/Modelo Global NL Controlador modulador de torque/Planta/Subsistema Electromagnetico ==
  v_qs : Inport
  v_ds : Inport  Port=2
  v_0s : Inport  Port=3
  ωm : Inport  Port=4
  R_s(T(t)) : Inport  Port=5
  Add : Sum  Inputs=-++
  Add1 : Sum  Inputs=--+
  Add2 : Sum  Inputs=|-+
  Add3 : Sum  Inputs=|++
  Gain : Gain  Gain=1/L_q
  Gain1 : Gain  Gain=1/L_d
  Gain2 : Gain  Gain=1/L_ls
  Gain3 : Gain  Gain=P_p
  Gain4 : Gain  Gain=L_d
  Gain5 : Gain  Gain=L_q
  Gain6 : Gain  Gain=3/2*P_p
  Gain7 : Gain  Gain=L_d-L_q
  Integrator : Integrator
  Integrator1 : Integrator  InitialCondition=i_ds_inicial
  Integrator2 : Integrator
  Product{,1..6} (7 alike) : Product
  Sum3 : Sum  Inputs=|++
  λ : Constant  Value=lambda_r
  i_qs : Outport
  i_ds : Outport  Port=2
  i_0s : Outport  Port=3
  T_m : Outport  Port=4
  wires:
  v_0s/1 -> Add2/2
  Gain5/1 -> Add/3
  Gain3/1 -> Product4/2, Product3/1  "ωr"
  Integrator/1 -> Product4/1, Product/2, i_qs/1, Product5/1, Product6/1
  v_qs/1 -> Add1/3
  R_s(T(t))/1 -> Product2/2, Product1/1, Product/1
  Gain4/1 -> Sum3/1
  Product1/1 -> Add/1
  Integrator2/1 -> i_0s/1, Product2/1
  Sum3/1 -> Product3/2
  Integrator1/1 -> Gain4/1, Product1/2, i_ds/1, Product6/2
  Product/1 -> Add1/2
  Product4/1 -> Gain5/1
  ωm/1 -> Gain3/1
  Add3/1 -> Gain6/1
  Gain/1 -> Integrator/1
  Gain6/1 -> T_m/1
  Product2/1 -> Add2/1
  λ/1 -> Sum3/2, Product5/2
  Gain1/1 -> Integrator1/1
  Add/1 -> Gain1/1
  Add1/1 -> Gain/1
  Product6/1 -> Gain7/1
  Product3/1 -> Add1/1
  Gain2/1 -> Integrator2/1
  Gain7/1 -> Add3/2
  v_ds/1 -> Add/2
  Add2/1 -> Gain2/1
  Product5/1 -> Add3/1

== system SistemaCompleto_PMSM/Modelo Global NL Controlador modulador de torque/Planta/Subsistema Mecanico ==
  Tld(t)[N.m] : Inport
  Tm(t)[N.m] : Inport  Port=2
  1/J_eq[kg.m2] : Gain  Gain=1/J_eq
  Gain : Gain  Gain=1/r
  Gain1 : Gain  Gain=1/r
  Integrator : Integrator  InitialCondition=pos_inicial*r
  Integrator1 : Integrator
  Sin : Trigonometry
  Sum : Sum  Inputs=-+-
  Sum1 : Sum
  "[N.m/rad]" : Gain  Gain=g*k_l
  b_eq[N.m/rad/s] : Gain  Gain=b_eq
  θm(t) : Outport
  ωm(t) : Outport  Port=2
  wires:
  Gain1/1 -> Sin/1
  Sin/1 -> "[N.m/rad]"/1  "θm[rad]"
  Integrator1/1 -> Integrator/1, ωm(t)/1, b_eq[N.m/rad/s]/1  "ωm[rad/s]"
  Tld(t)[N.m]/1 -> Sum1/1
  b_eq[N.m/rad/s]/1 -> Sum/3
  1/J_eq[kg.m2]/1 -> Integrator1/1  "dω/dt [rad/s^2]"
  Gain/1 -> Sum/1
  "[N.m/rad]"/1 -> Sum1/2
  Integrator/1 -> θm(t)/1, Gain1/1  "θm[rad]"
  Sum/1 -> 1/J_eq[kg.m2]/1
  Tm(t)[N.m]/1 -> Sum/2
  Sum1/1 -> Gain/1

== system SistemaCompleto_PMSM/Modelo Global NL Controlador modulador de torque/Planta/Subsistema Térmico ==
  i_qs2 : Inport
  i_ds2 : Inport  Port=2
  i_0s2 : Inport  Port=3
  Add : Sum  Inputs=+-
  Add1 : Sum
  Add2 : Sum  Inputs=+++
  Add3 : Sum  Inputs=+-
  Add4 : Sum  Inputs=-+
  Constant : Constant  Value=T_sREF
  Constant1 : Constant
  Constant2 : Constant  Value=T_amb
  Gain : Gain  Gain=R_sREF
  Gain1 : Gain  Gain=a_cu
  Gain2 : Gain  Gain=3/2
  Gain3 : Gain  Gain=2
  Gain4 : Gain  Gain=1/C_ts
  Gain5 : Gain  Gain=1/R_ts_amb
  Integrator : Integrator  InitialCondition=20
  Product : Product
  Square : Math  Operator=square  OutDataTypeStr=double
  Square1 : Math  Operator=square
  Square2 : Math  Operator=square
  R_s : Outport
  T_s : Outport  Port=2
  wires:
  Constant1/1 -> Add1/2
  Constant/1 -> Add/2
  i_qs2/1 -> Square/1
  Gain/1 -> R_s/1, Product/1
  Square/1 -> Add2/1
  Add2/1 -> Gain2/1
  Constant2/1 -> Add4/1
  i_ds2/1 -> Square1/1
  Gain5/1 -> Add3/2
  Integrator/1 -> Add4/2, T_s/1, Add/1  "T_s"
  Add1/1 -> Gain/1
  i_0s2/1 -> Square2/1
  Square1/1 -> Add2/2
  Product/1 -> Add3/1  "Ps_Perd"
  Gain2/1 -> Product/2
  Add/1 -> Gain1/1
  Square2/1 -> Gain3/1
  Gain1/1 -> Add1/1
  Add3/1 -> Gain4/1
  Add4/1 -> Gain5/1
  Gain3/1 -> Add2/3
  Gain4/1 -> Integrator/1

== system SistemaCompleto_PMSM/Modelo Global NL Controlador modulador de torque/Planta/TI de Park ==
  f_q : Inport
  f_d : Inport  Port=2
  f_0 : Inport  Port=3
  θ_r : Inport  Port=4
  Add : Sum  Inputs=+++
  Add1 : Sum  Inputs=+-
  Add2 : Sum
  Add3 : Sum  Inputs=+++
  Add4 : Sum  Inputs=+++
  Constant : Constant  Value=2/3*pi
  Constant1 : Constant  Value=2/3*pi
  Cos : Trigonometry  Operator=cos
  Cos1 : Trigonometry
  Cos2 : Trigonometry  Operator=cos
  Cos3 : Trigonometry  Operator=cos
  Cos4 : Trigonometry
  Cos5 : Trigonometry
  Product{,1..5} (6 alike) : Product
  f_a : Outport
  f_b : Outport  Port=2
  f_c : Outport  Port=3
  wires:
  Product4/1 -> Add3/2
  Cos1/1 -> Product1/1
  Cos/1 -> Product/1
  Product1/1 -> Add/2
  Add3/1 -> f_b/1
  Cos3/1 -> Product3/1
  Product3/1 -> Add3/1
  f_d/1 -> Product1/2, Product5/2, Product4/2
  Constant1/1 -> Add2/2
  Constant/1 -> Add1/2
  f_0/1 -> Add3/3, Add4/3, Add/3
  Add1/1 -> Cos3/1, Cos4/1
  Product/1 -> Add/1
  f_q/1 -> Product/2, Product2/2, Product3/2
  Cos4/1 -> Product4/1
  θ_r/1 -> Add2/1, Add1/1, Cos/1, Cos1/1
  Add/1 -> f_a/1
  Add4/1 -> f_c/1
  Cos2/1 -> Product2/1
  Cos5/1 -> Product5/1
  Add2/1 -> Cos5/1, Cos2/1
  Product2/1 -> Add4/1
  Product5/1 -> Add4/2

== system SistemaCompleto_PMSM/Modelo Global NL Controlador modulador de torque/Planta/Transformacion de Park ==
  f_a : Inport
  f_b : Inport  Port=2
  f_c : Inport  Port=3
  θ_r : Inport  Port=4
  Add : Sum  Inputs=+++
  Add1 : Sum  Inputs=+-
  Add2 : Sum
  Add3 : Sum  Inputs=+++
  Add4 : Sum  Inputs=+++
  Constant : Constant  Value=2/3*pi
  Constant1 : Constant  Value=2/3*pi
  Cos : Trigonometry  Operator=cos
  Cos1 : Trigonometry  Operator=cos
  Cos2 : Trigonometry  Operator=cos
  Cos3 : Trigonometry
  Cos4 : Trigonometry
  Cos5 : Trigonometry
  Gain1 : Gain  Gain=2/3
  Gain2 : Gain  Gain=2/3
  Gain3 : Gain  Gain=1/3
  Product{,1..5} (6 alike) : Product
  f_q : Outport
  f_d : Outport  Port=2
  f_0 : Outport  Port=3
  wires:
  Cos5/1 -> Product5/1
  Gain2/1 -> f_q/1
  Product5/1 -> Add3/3
  Add/1 -> Gain2/1
  θ_r/1 -> Cos3/1, Cos/1, Add1/1, Add2/1
  Cos4/1 -> Product4/1
  Cos2/1 -> Product2/1
  f_a/1 -> Add4/3, Product3/2, Product/2
  Product/1 -> Add/1
  Add1/1 -> Cos1/1, Cos4/1
  f_c/1 -> Product2/2, Product5/2, Add4/1
  Constant/1 -> Add1/2
  Constant1/1 -> Add2/2
  f_b/1 -> Product1/2, Product4/2, Add4/2
  Add2/1 -> Cos2/1, Cos5/1
  Add4/1 -> Gain3/1
  Product3/1 -> Add3/1
  Product2/1 -> Add/3
  Gain3/1 -> f_0/1
  Cos3/1 -> Product3/1
  Add3/1 -> Gain1/1
  Gain1/1 -> f_d/1
  Product1/1 -> Add/2
  Cos/1 -> Product/1
  Cos1/1 -> Product1/1
  Product4/1 -> Add3/2

== system SistemaCompleto_PMSM/Modelo Global NL Controlador modulador de torque1/Planta/Subsistema Electromagnetico ==
  v_qs : Inport
  v_ds : Inport  Port=2
  v_0s : Inport  Port=3
  ωm : Inport  Port=4
  R_s(T(t)) : Inport  Port=5
  Add : Sum  Inputs=-++
  Add1 : Sum  Inputs=--+
  Add2 : Sum  Inputs=|-+
  Add3 : Sum  Inputs=|++
  Gain : Gain  Gain=1/L_q
  Gain1 : Gain  Gain=1/L_d
  Gain2 : Gain  Gain=1/L_ls
  Gain3 : Gain  Gain=P_p
  Gain4 : Gain  Gain=L_d
  Gain5 : Gain  Gain=L_q
  Gain6 : Gain  Gain=3/2*P_p
  Gain7 : Gain  Gain=L_d-L_q
  Integrator : Integrator
  Integrator1 : Integrator  InitialCondition=i_ds_inicial
  Integrator2 : Integrator
  Product{,1..6} (7 alike) : Product
  Sum3 : Sum  Inputs=|++
  λ : Constant  Value=lambda_r
  i_qs : Outport
  i_ds : Outport  Port=2
  i_0s : Outport  Port=3
  T_m : Outport  Port=4
  wires:
  v_0s/1 -> Add2/2
  Gain5/1 -> Add/3
  Gain3/1 -> Product4/2, Product3/1  "ωr"
  Integrator/1 -> Product4/1, Product/2, i_qs/1, Product5/1, Product6/1
  v_qs/1 -> Add1/3
  R_s(T(t))/1 -> Product2/2, Product1/1, Product/1
  Gain4/1 -> Sum3/1
  Product1/1 -> Add/1
  Integrator2/1 -> i_0s/1, Product2/1
  Sum3/1 -> Product3/2
  Integrator1/1 -> Gain4/1, Product1/2, i_ds/1, Product6/2
  Product/1 -> Add1/2
  Product4/1 -> Gain5/1
  ωm/1 -> Gain3/1
  Add3/1 -> Gain6/1
  Gain/1 -> Integrator/1
  Gain6/1 -> T_m/1
  Product2/1 -> Add2/1
  λ/1 -> Sum3/2, Product5/2
  Gain1/1 -> Integrator1/1
  Add/1 -> Gain1/1
  Add1/1 -> Gain/1
  Product6/1 -> Gain7/1
  Product3/1 -> Add1/1
  Gain2/1 -> Integrator2/1
  Gain7/1 -> Add3/2
  v_ds/1 -> Add/2
  Add2/1 -> Gain2/1
  Product5/1 -> Add3/1

== system SistemaCompleto_PMSM/Modelo Global NL Controlador modulador de torque1/Planta/Subsistema Mecanico ==
  Tld(t)[N.m] : Inport
  Tm(t)[N.m] : Inport  Port=2
  1/J_eq[kg.m2] : Gain  Gain=1/J_eq
  Gain : Gain  Gain=1/r
  Gain1 : Gain  Gain=1/r
  Integrator : Integrator  InitialCondition=pos_inicial*r
  Integrator1 : Integrator
  Sin : Trigonometry
  Sum : Sum  Inputs=-+-
  Sum1 : Sum
  "[N.m/rad]" : Gain  Gain=g*k_l
  b_eq[N.m/rad/s] : Gain  Gain=b_eq
  θm(t) : Outport
  ωm(t) : Outport  Port=2
  wires:
  Gain1/1 -> Sin/1
  Sin/1 -> "[N.m/rad]"/1  "θm[rad]"
  Integrator1/1 -> Integrator/1, ωm(t)/1, b_eq[N.m/rad/s]/1  "ωm[rad/s]"
  Tld(t)[N.m]/1 -> Sum1/1
  b_eq[N.m/rad/s]/1 -> Sum/3
  1/J_eq[kg.m2]/1 -> Integrator1/1  "dω/dt [rad/s^2]"
  Gain/1 -> Sum/1
  "[N.m/rad]"/1 -> Sum1/2
  Integrator/1 -> θm(t)/1, Gain1/1  "θm[rad]"
  Sum/1 -> 1/J_eq[kg.m2]/1
  Tm(t)[N.m]/1 -> Sum/2
  Sum1/1 -> Gain/1

== system SistemaCompleto_PMSM/Modelo Global NL Controlador modulador de torque1/Planta/Subsistema Térmico ==
  i_qs2 : Inport
  i_ds2 : Inport  Port=2
  i_0s2 : Inport  Port=3
  Add : Sum  Inputs=+-
  Add1 : Sum
  Add2 : Sum  Inputs=+++
  Add3 : Sum  Inputs=+-
  Add4 : Sum  Inputs=-+
  Constant : Constant  Value=T_sREF
  Constant1 : Constant
  Constant2 : Constant  Value=T_amb
  Gain : Gain  Gain=R_sREF
  Gain1 : Gain  Gain=a_cu
  Gain2 : Gain  Gain=3/2
  Gain3 : Gain  Gain=2
  Gain4 : Gain  Gain=1/C_ts
  Gain5 : Gain  Gain=1/R_ts_amb
  Integrator : Integrator  InitialCondition=20
  Product : Product
  Square : Math  Operator=square  OutDataTypeStr=double
  Square1 : Math  Operator=square
  Square2 : Math  Operator=square
  R_s : Outport
  T_s : Outport  Port=2
  wires:
  Constant1/1 -> Add1/2
  Constant/1 -> Add/2
  i_qs2/1 -> Square/1
  Gain/1 -> R_s/1, Product/1
  Square/1 -> Add2/1
  Add2/1 -> Gain2/1
  Constant2/1 -> Add4/1
  i_ds2/1 -> Square1/1
  Gain5/1 -> Add3/2
  Integrator/1 -> Add4/2, T_s/1, Add/1  "T_s"
  Add1/1 -> Gain/1
  i_0s2/1 -> Square2/1
  Square1/1 -> Add2/2
  Product/1 -> Add3/1  "Ps_Perd"
  Gain2/1 -> Product/2
  Add/1 -> Gain1/1
  Square2/1 -> Gain3/1
  Gain1/1 -> Add1/1
  Add3/1 -> Gain4/1
  Add4/1 -> Gain5/1
  Gain3/1 -> Add2/3
  Gain4/1 -> Integrator/1

== system SistemaCompleto_PMSM/Modelo Global NL Controlador modulador de torque1/Planta/TI de Park ==
  f_q : Inport
  f_d : Inport  Port=2
  f_0 : Inport  Port=3
  θ_r : Inport  Port=4
  Add : Sum  Inputs=+++
  Add1 : Sum  Inputs=+-
  Add2 : Sum
  Add3 : Sum  Inputs=+++
  Add4 : Sum  Inputs=+++
  Constant : Constant  Value=2/3*pi
  Constant1 : Constant  Value=2/3*pi
  Cos : Trigonometry  Operator=cos
  Cos1 : Trigonometry
  Cos2 : Trigonometry  Operator=cos
  Cos3 : Trigonometry  Operator=cos
  Cos4 : Trigonometry
  Cos5 : Trigonometry
  Product{,1..5} (6 alike) : Product
  f_a : Outport
  f_b : Outport  Port=2
  f_c : Outport  Port=3
  wires:
  Product4/1 -> Add3/2
  Cos1/1 -> Product1/1
  Cos/1 -> Product/1
  Product1/1 -> Add/2
  Add3/1 -> f_b/1
  Cos3/1 -> Product3/1
  Product3/1 -> Add3/1
  f_d/1 -> Product1/2, Product5/2, Product4/2
  Constant1/1 -> Add2/2
  Constant/1 -> Add1/2
  f_0/1 -> Add3/3, Add4/3, Add/3
  Add1/1 -> Cos3/1, Cos4/1
  Product/1 -> Add/1
  f_q/1 -> Product/2, Product2/2, Product3/2
  Cos4/1 -> Product4/1
  θ_r/1 -> Add2/1, Add1/1, Cos/1, Cos1/1
  Add/1 -> f_a/1
  Add4/1 -> f_c/1
  Cos2/1 -> Product2/1
  Cos5/1 -> Product5/1
  Add2/1 -> Cos5/1, Cos2/1
  Product2/1 -> Add4/1
  Product5/1 -> Add4/2

== system SistemaCompleto_PMSM/Modelo Global NL Controlador modulador de torque1/Planta/Transformacion de Park ==
  f_a : Inport
  f_b : Inport  Port=2
  f_c : Inport  Port=3
  θ_r : Inport  Port=4
  Add : Sum  Inputs=+++
  Add1 : Sum  Inputs=+-
  Add2 : Sum
  Add3 : Sum  Inputs=+++
  Add4 : Sum  Inputs=+++
  Constant : Constant  Value=2/3*pi
  Constant1 : Constant  Value=2/3*pi
  Cos : Trigonometry  Operator=cos
  Cos1 : Trigonometry  Operator=cos
  Cos2 : Trigonometry  Operator=cos
  Cos3 : Trigonometry
  Cos4 : Trigonometry
  Cos5 : Trigonometry
  Gain1 : Gain  Gain=2/3
  Gain2 : Gain  Gain=2/3
  Gain3 : Gain  Gain=1/3
  Product{,1..5} (6 alike) : Product
  f_q : Outport
  f_d : Outport  Port=2
  f_0 : Outport  Port=3
  wires:
  Cos5/1 -> Product5/1
  Gain2/1 -> f_q/1
  Product5/1 -> Add3/3
  Add/1 -> Gain2/1
  θ_r/1 -> Cos3/1, Cos/1, Add1/1, Add2/1
  Cos4/1 -> Product4/1
  Cos2/1 -> Product2/1
  f_a/1 -> Add4/3, Product3/2, Product/2
  Product/1 -> Add/1
  Add1/1 -> Cos1/1, Cos4/1
  f_c/1 -> Product2/2, Product5/2, Add4/1
  Constant/1 -> Add1/2
  Constant1/1 -> Add2/2
  f_b/1 -> Product1/2, Product4/2, Add4/2
  Add2/1 -> Cos2/1, Cos5/1
  Add4/1 -> Gain3/1
  Product3/1 -> Add3/1
  Product2/1 -> Add/3
  Gain3/1 -> f_0/1
  Cos3/1 -> Product3/1
  Add3/1 -> Gain1/1
  Gain1/1 -> f_d/1
  Product1/1 -> Add/2
  Cos/1 -> Product/1
  Cos1/1 -> Product1/1
  Product4/1 -> Add3/2
